simulink model "Sensors_UltraStick25e"  (R2016b)
settings: Solver=VariableStepAuto  StartTime=0.0  StopTime=10.0  RelTol=1e-3
undefined symbols (not defined in the file or in its folder): AC
libraries: Sensors_Lib x13
settings Model: Creator=UAVLAB  LastModifiedBy=UAVLAB

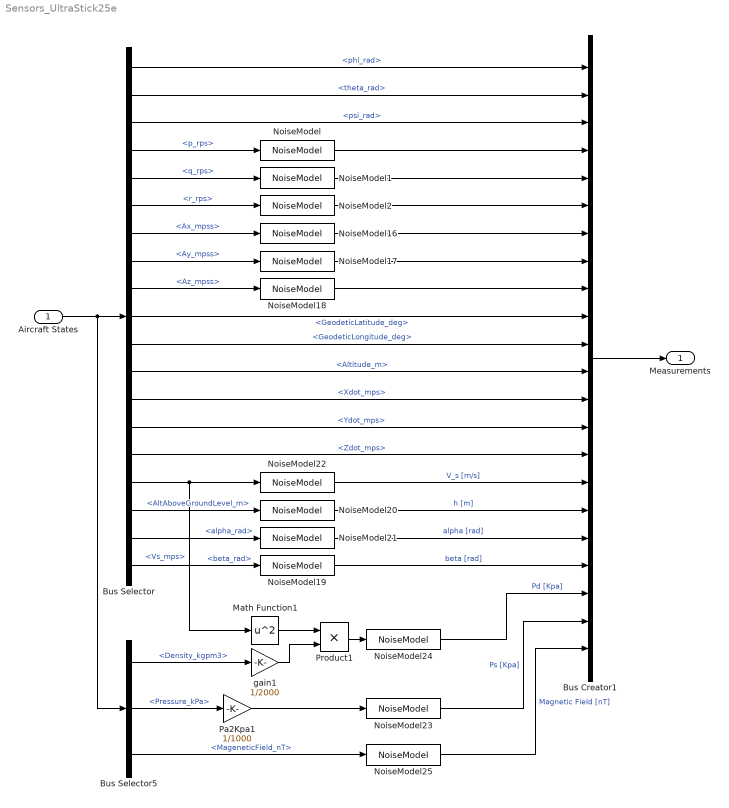
== system Sensors_UltraStick25e ==
  Aircraft States : Inport  OutDataTypeStr=Bus: States
  Bus Creator1 : BusCreator  Inputs=22  OutDataTypeStr=Bus: Sensors
      settings: InheritFromInputs=off
  Bus Selector : BusSelector  OutputSignals=RigidStates.Euler.phi_rad,RigidStates.Euler.theta_rad,RigidStates.Euler.psi_rad,RigidStates.AngVel.p_rps,RigidStates.AngVel.q_rps,RigidStates.AngVel.r_rps,RigidStates.Accels.Ax_mpss,RigidStates.Accels.Ay_mpss,RigidStates.Accels.Az_mpss,AuxVar.Nav.GeodeticLatitude_deg,AuxVar.Nav.GeodeticLongitude_deg,AuxVar.Nav.Altitude_m,AuxVar.V_e.Xdot_mps,AuxVar.V_e.Ydot_mps,AuxVar.V_e.Zdot_mps,AuxVar.WindAxesParams.Vs_mps,AuxVar.Nav.AltAboveGroundLevel_m,AuxVar.WindAxesParams.alpha_rad,AuxVar.WindAxesParams.beta_rad
  Bus Selector5 : BusSelector  OutputSignals=EnvData.Density_kgpm3,EnvData.Pressure_kPa,EnvData.MageneticField_nT
  Math Function1 : Math  Operator=square  SaturateOnIntegerOverflow=on
  NoiseModel : Sensors_Lib/NoiseModel  noise_on=AC.Sensors.NoiseOn  sigma=AC.Sensors.IMU.p_noise  seed=878230  bias=AC.Sensors.IMU.p_bias  scf=AC.Sensors.IMU.p_scf  timestep=SampleTime
  NoiseModel1 : Sensors_Lib/NoiseModel  noise_on=AC.Sensors.NoiseOn  sigma=AC.Sensors.IMU.p_noise  seed=878230  bias=AC.Sensors.IMU.p_bias  scf=AC.Sensors.IMU.p_scf  timestep=SampleTime
  NoiseModel16 : Sensors_Lib/NoiseModel  noise_on=AC.Sensors.NoiseOn  sigma=AC.Sensors.IMU.ax_noise  seed=878233  bias=AC.Sensors.IMU.ax_bias  scf=AC.Sensors.IMU.ax_scf  timestep=SampleTime
  NoiseModel17 : Sensors_Lib/NoiseModel  noise_on=AC.Sensors.NoiseOn  sigma=AC.Sensors.IMU.ay_noise  seed=878234  bias=AC.Sensors.IMU.ay_bias  scf=AC.Sensors.IMU.ay_scf  timestep=SampleTime
  NoiseModel18 : Sensors_Lib/NoiseModel  noise_on=AC.Sensors.NoiseOn  sigma=AC.Sensors.IMU.az_noise  seed=878235  bias=AC.Sensors.IMU.az_bias  scf=AC.Sensors.IMU.az_scf  timestep=SampleTime
  NoiseModel19 : Sensors_Lib/NoiseModel  noise_on=AC.Sensors.NoiseOn  sigma=AC.Sensors.AirData.beta_noise  seed=87828  bias=AC.Sensors.AirData.beta_bias  scf=AC.Sensors.AirData.beta_scf  timestep=SampleTime
  NoiseModel2 : Sensors_Lib/NoiseModel  noise_on=AC.Sensors.NoiseOn  sigma=AC.Sensors.IMU.r_noise  seed=878230  bias=AC.Sensors.IMU.r_bias  scf=AC.Sensors.IMU.r_scf  timestep=SampleTime
  NoiseModel20 : Sensors_Lib/NoiseModel  noise_on=AC.Sensors.NoiseOn  sigma=AC.Sensors.AirData.h_noise  seed=87828  bias=AC.Sensors.AirData.h_bias  scf=AC.Sensors.AirData.h_scf  timestep=SampleTime
  NoiseModel21 : Sensors_Lib/NoiseModel  noise_on=AC.Sensors.NoiseOn  sigma=AC.Sensors.AirData.alpha_noise  seed=87828  bias=AC.Sensors.AirData.alpha_bias  scf=AC.Sensors.AirData.alpha_scf  timestep=SampleTime
  NoiseModel22 : Sensors_Lib/NoiseModel  noise_on=AC.Sensors.NoiseOn  sigma=AC.Sensors.AirData.ias_noise  seed=878236  bias=AC.Sensors.AirData.ias_bias  scf=AC.Sensors.AirData.ias_scf  timestep=SampleTime
  NoiseModel23 : Sensors_Lib/NoiseModel  noise_on=AC.Sensors.NoiseOn  sigma=AC.Sensors.AirData.Ps_noise  seed=8782378  bias=AC.Sensors.AirData.Ps_bias  scf=AC.Sensors.AirData.Ps_scf  timestep=SampleTime
  NoiseModel24 : Sensors_Lib/NoiseModel  noise_on=AC.Sensors.NoiseOn  sigma=AC.Sensors.AirData.Pd_noise  seed=87823  bias=AC.Sensors.AirData.Pd_bias  scf=AC.Sensors.AirData.Pd_scf  timestep=SampleTime
  NoiseModel25 : Sensors_Lib/NoiseModel  noise_on=AC.Sensors.NoiseOn  sigma=[AC.Sensors.IMU.hx_noise, AC.Sensors.IMU.hy_noise,AC.Sensors.IMU.hz_noise]  seed=878237  bias=[AC.Sensors.IMU.hx_bias, AC.Sensors.IMU.hy_bias, AC.Sensors.IMU.hz_bias]  scf=[AC.Sensors.IMU.hx_scf, AC.Sensors.IMU.hy_scf, AC.Sensors.IMU.hz_scf]  timestep=SampleTime
  Pa2Kpa1 : Gain  Gain=1/1000
  Product1 : Product  RndMeth=Zero
  gain1 : Gain  Gain=1/2000
  Measurements : Outport  OutDataTypeStr=Bus: Sensors
  wires:
  Aircraft States/1 -> Bus Selector5/1, Bus Selector/1
  Bus Selector/1 -> Bus Creator1/1  "<phi_rad>"
  Bus Selector/2 -> Bus Creator1/2  "<theta_rad>"
  Bus Creator1/1 -> Measurements/1
  Bus Selector/4 -> NoiseModel/1  "<p_rps>"
  Bus Selector/5 -> NoiseModel1/1  "<q_rps>"
  Bus Selector/6 -> NoiseModel2/1  "<r_rps>"
  NoiseModel/1 -> Bus Creator1/4
  NoiseModel1/1 -> Bus Creator1/5
  NoiseModel2/1 -> Bus Creator1/6
  Bus Selector/7 -> NoiseModel16/1  "<Ax_mpss>"
  Bus Selector/8 -> NoiseModel17/1  "<Ay_mpss>"
  Bus Selector/9 -> NoiseModel18/1  "<Az_mpss>"
  Bus Selector/3 -> Bus Creator1/3  "<psi_rad>"
  NoiseModel18/1 -> Bus Creator1/9
  NoiseModel16/1 -> Bus Creator1/7
  NoiseModel17/1 -> Bus Creator1/8
  Bus Selector/11 -> Bus Creator1/11  "<GeodeticLongitude_deg>"
  Bus Selector/17 -> NoiseModel20/1  "<AltAboveGroundLevel_m>"
  Bus Selector/18 -> NoiseModel21/1  "<alpha_rad>"
  Bus Selector/19 -> NoiseModel19/1  "<beta_rad>"
  Bus Selector/10 -> Bus Creator1/10  "<GeodeticLatitude_deg>"
  Bus Selector/12 -> Bus Creator1/12  "<Altitude_m>"
  Bus Selector/13 -> Bus Creator1/13  "<Xdot_mps>"
  Bus Selector/14 -> Bus Creator1/14  "<Ydot_mps>"
  Bus Selector/15 -> Bus Creator1/15  "<Zdot_mps>"
  NoiseModel22/1 -> Bus Creator1/16  "V_s [m/s]"
  NoiseModel20/1 -> Bus Creator1/17  "h [m]"
  NoiseModel21/1 -> Bus Creator1/18  "alpha [rad]"
  NoiseModel19/1 -> Bus Creator1/19  "beta [rad]"
  Bus Selector/16 -> Math Function1/1, NoiseModel22/1  "<Vs_mps>"
  NoiseModel25/1 -> Bus Creator1/22  "Magnetic Field [nT]"
  NoiseModel23/1 -> Bus Creator1/21  "Ps [Kpa]"
  NoiseModel24/1 -> Bus Creator1/20  "Pd [Kpa]"
  Product1/1 -> NoiseModel24/1
  gain1/1 -> Product1/2
  Math Function1/1 -> Product1/1
  Bus Selector5/1 -> gain1/1  "<Density_kgpm3>"
  Pa2Kpa1/1 -> NoiseModel23/1
  Bus Selector5/2 -> Pa2Kpa1/1  "<Pressure_kPa>"
  Bus Selector5/3 -> NoiseModel25/1  "<MageneticField_nT>"
